simulink model "BenchmarkModel_Dynamic_TestCase"  (R2020a)
settings: Solver=ode45  StartTime=0.0  StopTime=5  RelTol=1e-3
undefined symbols (not defined in the file): Angle, D1, Delta, find_system, Magnitude
libraries: powerlib x91, powerlib_meascontrol x31, simulink x6, dspsrcs4 x3, dspsigops x2, sps_avr x1
(part 3 of 3)

== system BenchmarkModel_Dynamic_TestCase/VSI Converter1/Current Control/PLL & Park Transformation/Filter2 ==
  in : Inport
  Demux : Demux  Outputs=3
  Mux : Mux  Inputs=3
  Transfer Fcn1 : TransferFcn  Denominator=[1/(2*pi*Ft) 1]
  Transfer Fcn2 : TransferFcn  Denominator=[1/(2*pi*Ft) 1]
  Transfer Fcn3 : TransferFcn  Denominator=[1/(2*pi*Ft) 1]
  out : Outport  VectorParamsAs1DForOutWhenUnconnected=off
  wires:
  Mux/1 -> out/1
  in/1 -> Demux/1
  Transfer Fcn3/1 -> Mux/3
  Transfer Fcn2/1 -> Mux/2
  Transfer Fcn1/1 -> Mux/1
  Demux/3 -> Transfer Fcn3/1
  Demux/1 -> Transfer Fcn1/1
  Demux/2 -> Transfer Fcn2/1

== system BenchmarkModel_Dynamic_TestCase/VSI Converter1/Current Control/PLL & Park Transformation/Filter3 ==
  in : Inport
  Demux : Demux  Outputs=3
  Mux : Mux  Inputs=3
  Transfer Fcn1 : TransferFcn  Denominator=[1/(2*pi*Ft) 1]
  Transfer Fcn2 : TransferFcn  Denominator=[1/(2*pi*Ft) 1]
  Transfer Fcn3 : TransferFcn  Denominator=[1/(2*pi*Ft) 1]
  out : Outport  VectorParamsAs1DForOutWhenUnconnected=off
  wires:
  Demux/2 -> Transfer Fcn2/1
  Demux/1 -> Transfer Fcn1/1
  Demux/3 -> Transfer Fcn3/1
  Transfer Fcn1/1 -> Mux/1
  Transfer Fcn2/1 -> Mux/2
  Transfer Fcn3/1 -> Mux/3
  in/1 -> Demux/1
  Mux/1 -> out/1

== system BenchmarkModel_Dynamic_TestCase/VSI Converter1/Current Control/PLL & Park Transformation/MAF-PLL ==
  note: MAF
  Vabc : Inport
  Autoresettable integral theta : Subsystem
  Constant : Constant  Value=Non_limited_theta
  Demux9 : Demux  Outputs=2
  Divide : Product  Inputs=*/
  Gain : Gain  Gain=1/(2*pi)
  Gain1 : Gain  Gain=2*pi
  Gain2 : Gain  Gain=Ki_PLL
  Integrator : Integrator
  MAF : Subsystem
  MAF1 : Subsystem
  Proportional gain : Gain  Gain=Kp_PLL
  Selector : Selector  InputPortWidth=3  IndexOptions=Index vector (dialog)  Indices=[2 1]  OutputSizes=1
  Sum : Sum  Inputs=++|
  Sum2 : Sum  Inputs=++|
  Switch : Switch  Criteria=u2 > Threshold
  abc to dq3 : powerlib_meascontrol/Transformations/abc to dq0  Alignment=90 degrees behind phase A axis
  integration of pulse : Integrator  InitialCondition=initPhase*pi/180
  nominal frequency : Constant  Value=initFreq
  Estimated Theta : Outport  VectorParamsAs1DForOutWhenUnconnected=off
  Estimated Frequency : Outport  Port=2  VectorParamsAs1DForOutWhenUnconnected=off
  wires:
  Autoresettable integral theta/1(Out1) -> Switch/3
  Switch/1 -> abc to dq3/2, Estimated Theta/1  "Theta_o"
  Constant/1 -> Switch/2
  MAF1/1(Output) -> Divide/2
  MAF/1(Output) -> Divide/1
  Gain1/1 -> Sum2/1
  Gain/1 -> Estimated Frequency/1
  Demux9/1 -> MAF/1(Input)  "Vq"
  Demux9/2 -> MAF1/1(Input)  "Vd"
  Divide/1 -> Gain2/1, Proportional gain/1
  Proportional gain/1 -> Sum/2  "Delta_W_o"
  integration of pulse/1 -> Switch/1  "Theta_o"
  Vabc/1 -> abc to dq3/1
  Selector/1 -> Demux9/1  "Vq,Vd"
  nominal frequency/1 -> Gain1/1
  Sum/1 -> Gain/1, integration of pulse/1, Autoresettable integral theta/1(In1)  "W_o"
  abc to dq3/1 -> Selector/1
  Gain2/1 -> Integrator/1
  Integrator/1 -> Sum2/2
  Sum2/1 -> Sum/1

== system BenchmarkModel_Dynamic_TestCase/VSI Converter1/Current Control/PLL & Park Transformation/Park Capacitor Voltage ==
  note: PARK
  abc quantity : Inport
  f : Inport  Port=2
  Theta : Inport  Port=3
  Demux8 : Demux  Outputs=3
  Mag correction4 : Subsystem
  Phase correction4 : Subsystem
  Product : Product  Inputs=**
  Sum1 : Sum  Inputs=|+-
  Terminator7 : Terminator
  abc to dq7 : powerlib_meascontrol/Transformations/abc to dq0  Alignment=90 degrees behind phase A axis
  d quantity : Outport  VectorParamsAs1DForOutWhenUnconnected=off
  q quantity : Outport  Port=2  VectorParamsAs1DForOutWhenUnconnected=off
  wires:
  Phase correction4/1(Out1) -> Sum1/2
  f/1 -> Phase correction4/1(freq), Mag correction4/1(freq)
  abc quantity/1 -> Product/1
  Product/1 -> abc to dq7/1
  Mag correction4/1(Out1) -> Product/2
  Demux8/3 -> Terminator7/1
  Theta/1 -> Sum1/1
  Sum1/1 -> abc to dq7/2
  Demux8/2 -> q quantity/1  "q"
  Demux8/1 -> d quantity/1  "d"
  abc to dq7/1 -> Demux8/1

== system BenchmarkModel_Dynamic_TestCase/VSI Converter1/Current Control/PLL & Park Transformation/Park Current ==
  note: PARK
  abc quantity : Inport
  f : Inport  Port=2
  Theta : Inport  Port=3
  Demux8 : Demux  Outputs=3
  Mag correction4 : Subsystem
  Phase correction4 : Subsystem
  Product : Product  Inputs=**
  Sum1 : Sum  Inputs=|+-
  Terminator7 : Terminator
  abc to dq7 : powerlib_meascontrol/Transformations/abc to dq0  Alignment=90 degrees behind phase A axis
  d quantity : Outport  VectorParamsAs1DForOutWhenUnconnected=off
  q quantity : Outport  Port=2  VectorParamsAs1DForOutWhenUnconnected=off
  wires:
  Phase correction4/1(Out1) -> Sum1/2
  f/1 -> Phase correction4/1(freq), Mag correction4/1(freq)
  abc quantity/1 -> Product/1
  Product/1 -> abc to dq7/1
  Mag correction4/1(Out1) -> Product/2
  Demux8/3 -> Terminator7/1
  Theta/1 -> Sum1/1
  Sum1/1 -> abc to dq7/2
  Demux8/2 -> q quantity/1  "q"
  Demux8/1 -> d quantity/1  "d"
  abc to dq7/1 -> Demux8/1

== system BenchmarkModel_Dynamic_TestCase/VSI Converter1/Current Control/PLL & Park Transformation/Park Grid Voltage ==
  note: PARK
  abc quantity : Inport
  f : Inport  Port=2
  Theta : Inport  Port=3
  Demux8 : Demux  Outputs=3
  Mag correction4 : Subsystem
  Phase correction4 : Subsystem
  Product : Product  Inputs=**
  Sum1 : Sum  Inputs=|+-
  Terminator7 : Terminator
  abc to dq7 : powerlib_meascontrol/Transformations/abc to dq0  Alignment=90 degrees behind phase A axis
  d quantity : Outport  VectorParamsAs1DForOutWhenUnconnected=off
  q quantity : Outport  Port=2  VectorParamsAs1DForOutWhenUnconnected=off
  wires:
  abc to dq7/1 -> Demux8/1
  Demux8/1 -> d quantity/1  "d"
  Demux8/2 -> q quantity/1  "q"
  Sum1/1 -> abc to dq7/2
  Theta/1 -> Sum1/1
  Demux8/3 -> Terminator7/1
  Mag correction4/1(Out1) -> Product/2
  Product/1 -> abc to dq7/1
  abc quantity/1 -> Product/1
  f/1 -> Mag correction4/1(freq), Phase correction4/1(freq)
  Phase correction4/1(Out1) -> Sum1/2

== system BenchmarkModel_Dynamic_TestCase/VSI Converter1/Current Control/PLL & Park Transformation/concatenate//fase1 ==
  note: Vab
  note: Vbc
  note: Vca
  note: 3Va
  note: 3Vb
  note: 3Vc
  ab_bc_ca : Inport
  Add : Sum  Inputs=+-
  Add1 : Sum  Inputs=+-
  Add2 : Sum  Inputs=+-
  Demux : Demux  Outputs=3
  Gain : Gain  Gain=1/3
  Mux : Mux  Inputs=3
  a_b_c : Outport  VectorParamsAs1DForOutWhenUnconnected=off
  wires:
  Demux/2 -> Add1/1, Add2/2
  Demux/3 -> Add/2, Add2/1
  Demux/1 -> Add1/2, Add/1
  Gain/1 -> a_b_c/1
  Mux/1 -> Gain/1
  Add2/1 -> Mux/3
  Add1/1 -> Mux/2
  Add/1 -> Mux/1
  ab_bc_ca/1 -> Demux/1

== system BenchmarkModel_Dynamic_TestCase/VSI Converter1/Current Control/PLL & Park Transformation/concatenate//fase2 ==
  note: 3Vc
  note: 3Vb
  note: 3Va
  note: Vca
  note: Vbc
  note: Vab
  ab_bc_ca : Inport
  Add : Sum  Inputs=+-
  Add1 : Sum  Inputs=+-
  Add2 : Sum  Inputs=+-
  Demux : Demux  Outputs=3
  Gain : Gain  Gain=1/3
  Mux : Mux  Inputs=3
  a_b_c : Outport  VectorParamsAs1DForOutWhenUnconnected=off
  wires:
  ab_bc_ca/1 -> Demux/1
  Add/1 -> Mux/1
  Add1/1 -> Mux/2
  Add2/1 -> Mux/3
  Mux/1 -> Gain/1
  Gain/1 -> a_b_c/1
  Demux/1 -> Add/1, Add1/2
  Demux/3 -> Add2/1, Add/2
  Demux/2 -> Add2/2, Add1/1

== system BenchmarkModel_Dynamic_TestCase/VSI Converter1/Current Control/Qref --> Iqref/Parameter ==
  Constant8 : Constant  Value=1e-3
  Constant9 : Constant  Value=Cf
  Mux1 : Mux  Inputs=2
  Parameters : Outport  VectorParamsAs1DForOutWhenUnconnected=off
  wires:
  Mux1/1 -> Parameters/1
  Constant8/1 -> Mux1/1
  Constant9/1 -> Mux1/2

== system BenchmarkModel_Dynamic_TestCase/VSI Converter1/Current Control/Qref --> Iqref/Vc ==
  VCd : Inport
  VCq : Inport  Port=2
  Complex to Magnitude-Angle3 : ComplexToMagnitudeAngle
  Constant12 : Constant  Value=sqrt(2)
  Divide5 : Product  Inputs=*/
  Real-Imag to Complex3 : RealImagToComplex
  Terminator6 : Terminator
  Vc_rms : Outport  VectorParamsAs1DForOutWhenUnconnected=off
  wires:
  Real-Imag to Complex3/1 -> Complex to Magnitude-Angle3/1
  Complex to Magnitude-Angle3/2 -> Terminator6/1
  VCd/1 -> Real-Imag to Complex3/1
  VCq/1 -> Real-Imag to Complex3/2
  Constant12/1 -> Divide5/2
  Complex to Magnitude-Angle3/1 -> Divide5/1
  Divide5/1 -> Vc_rms/1

== system BenchmarkModel_Dynamic_TestCase/Subsystem/Three-Phase Tap Changer Transformer Pn MVA, Up // Us kV/Tap Changer Control/Edge Detector/NEGATIVE Edge ==
  IN : Inport
  IN previous : Inport  Port=2
  Enable : EnablePort  PropagateVarSize=During execution
  Relational Operator1 : RelationalOperator  Operator=>  RndMeth=Nearest  InputSameDT=on
  OUT : Outport  VectorParamsAs1DForOutWhenUnconnected=off
  wires:
  Relational Operator1/1 -> OUT/1
  IN previous/1 -> Relational Operator1/1
  IN/1 -> Relational Operator1/2

== system BenchmarkModel_Dynamic_TestCase/Subsystem/Three-Phase Tap Changer Transformer Pn MVA, Up // Us kV/Tap Changer Control/Edge Detector/POSITIVE Edge ==
  IN : Inport
  IN previous : Inport  Port=2
  Enable : EnablePort  PropagateVarSize=During execution
  Relational Operator1 : RelationalOperator  Operator=>  RndMeth=Nearest  InputSameDT=on
  OUT : Outport  VectorParamsAs1DForOutWhenUnconnected=off
  wires:
  Relational Operator1/1 -> OUT/1
  IN previous/1 -> Relational Operator1/2
  IN/1 -> Relational Operator1/1

== system BenchmarkModel_Dynamic_TestCase/VSI Converter1/Current Control/PLL & Park Transformation/MAF-PLL/Autoresettable integral theta ==
  In1 : Inport
  Add : Sum  Inputs=+-
  Constant : Constant  Value=2*pi
  Divide : Product  Inputs=*/  OutDataTypeStr=int32  SaturateOnIntegerOverflow=on
  Gain : Gain  Gain=2*pi
  Integrator : Integrator  InitialCondition=initPhase*pi/180
  Out1 : Outport  VectorParamsAs1DForOutWhenUnconnected=off
  wires:
  Add/1 -> Out1/1
  Gain/1 -> Add/2
  Divide/1 -> Gain/1
  Constant/1 -> Divide/2
  In1/1 -> Integrator/1
  Integrator/1 -> Divide/1, Add/1

== system BenchmarkModel_Dynamic_TestCase/VSI Converter1/Current Control/PLL & Park Transformation/MAF-PLL/MAF ==
  Input : Inport
  Delay of Tw : TransportDelay  DelayTime=Tw
  Gain : Gain  Gain=1/Tw
  Integrator2 : Integrator
  Sum : Sum  Inputs=+-
  Output : Outport  VectorParamsAs1DForOutWhenUnconnected=off
  wires:
  Integrator2/1 -> Output/1
  Delay of Tw/1 -> Sum/2
  Input/1 -> Sum/1, Delay of Tw/1
  Sum/1 -> Gain/1
  Gain/1 -> Integrator2/1

== system BenchmarkModel_Dynamic_TestCase/VSI Converter1/Current Control/PLL & Park Transformation/MAF-PLL/MAF1 ==
  Input : Inport
  Delay of Tw : TransportDelay  DelayTime=Tw
  Gain : Gain  Gain=1/Tw
  Integrator2 : Integrator  InitialCondition=326
  Sum : Sum  Inputs=+-
  Output : Outport  VectorParamsAs1DForOutWhenUnconnected=off
  wires:
  Gain/1 -> Integrator2/1
  Sum/1 -> Gain/1
  Input/1 -> Delay of Tw/1, Sum/1
  Delay of Tw/1 -> Sum/2
  Integrator2/1 -> Output/1

== system BenchmarkModel_Dynamic_TestCase/VSI Converter1/Current Control/PLL & Park Transformation/Park Capacitor Voltage/Mag correction4 ==
  freq : Inport
  Complex to Magnitude-Angle : ComplexToMagnitudeAngle
  Divide5 : Product  Inputs=**/
  Real-Imag to Complex : RealImagToComplex
  Terminator : Terminator
  w10 : Constant  Value=2*pi*Ft
  w11 : Constant
  w9 : Constant  Value=2*pi
  Out1 : Outport  VectorParamsAs1DForOutWhenUnconnected=off
  wires:
  freq/1 -> Divide5/2
  w10/1 -> Divide5/3
  w9/1 -> Divide5/1
  Divide5/1 -> Real-Imag to Complex/2
  Complex to Magnitude-Angle/2 -> Terminator/1
  Complex to Magnitude-Angle/1 -> Out1/1
  w11/1 -> Real-Imag to Complex/1
  Real-Imag to Complex/1 -> Complex to Magnitude-Angle/1

== system BenchmarkModel_Dynamic_TestCase/VSI Converter1/Current Control/PLL & Park Transformation/Park Capacitor Voltage/Phase correction4 ==
  freq : Inport
  Divide2 : Product  Inputs=**/
  Trigonometric Function1 : Trigonometry  Operator=atan
  w3 : Constant  Value=2*pi
  w4 : Constant  Value=2*pi*Ft
  Out1 : Outport  VectorParamsAs1DForOutWhenUnconnected=off
  wires:
  Trigonometric Function1/1 -> Out1/1
  Divide2/1 -> Trigonometric Function1/1
  freq/1 -> Divide2/2
  w4/1 -> Divide2/3
  w3/1 -> Divide2/1

== system BenchmarkModel_Dynamic_TestCase/VSI Converter1/Current Control/PLL & Park Transformation/Park Current/Mag correction4 ==
  freq : Inport
  Complex to Magnitude-Angle : ComplexToMagnitudeAngle
  Divide5 : Product  Inputs=**/
  Real-Imag to Complex : RealImagToComplex
  Terminator : Terminator
  w10 : Constant  Value=2*pi*Ft
  w11 : Constant
  w9 : Constant  Value=2*pi
  Out1 : Outport  VectorParamsAs1DForOutWhenUnconnected=off
  wires:
  freq/1 -> Divide5/2
  w10/1 -> Divide5/3
  w9/1 -> Divide5/1
  Divide5/1 -> Real-Imag to Complex/2
  Complex to Magnitude-Angle/2 -> Terminator/1
  Complex to Magnitude-Angle/1 -> Out1/1
  w11/1 -> Real-Imag to Complex/1
  Real-Imag to Complex/1 -> Complex to Magnitude-Angle/1

== system BenchmarkModel_Dynamic_TestCase/VSI Converter1/Current Control/PLL & Park Transformation/Park Current/Phase correction4 ==
  freq : Inport
  Divide2 : Product  Inputs=**/
  Trigonometric Function1 : Trigonometry  Operator=atan
  w3 : Constant  Value=2*pi
  w4 : Constant  Value=2*pi*Ft
  Out1 : Outport  VectorParamsAs1DForOutWhenUnconnected=off
  wires:
  Trigonometric Function1/1 -> Out1/1
  Divide2/1 -> Trigonometric Function1/1
  freq/1 -> Divide2/2
  w4/1 -> Divide2/3
  w3/1 -> Divide2/1

== system BenchmarkModel_Dynamic_TestCase/VSI Converter1/Current Control/PLL & Park Transformation/Park Grid Voltage/Mag correction4 ==
  freq : Inport
  Complex to Magnitude-Angle : ComplexToMagnitudeAngle
  Divide5 : Product  Inputs=**/
  Real-Imag to Complex : RealImagToComplex
  Terminator : Terminator
  w10 : Constant  Value=2*pi*Ft
  w11 : Constant
  w9 : Constant  Value=2*pi
  Out1 : Outport  VectorParamsAs1DForOutWhenUnconnected=off
  wires:
  Real-Imag to Complex/1 -> Complex to Magnitude-Angle/1
  w11/1 -> Real-Imag to Complex/1
  Complex to Magnitude-Angle/1 -> Out1/1
  Complex to Magnitude-Angle/2 -> Terminator/1
  Divide5/1 -> Real-Imag to Complex/2
  w9/1 -> Divide5/1
  w10/1 -> Divide5/3
  freq/1 -> Divide5/2

== system BenchmarkModel_Dynamic_TestCase/VSI Converter1/Current Control/PLL & Park Transformation/Park Grid Voltage/Phase correction4 ==
  freq : Inport
  Divide2 : Product  Inputs=**/
  Trigonometric Function1 : Trigonometry  Operator=atan
  w3 : Constant  Value=2*pi
  w4 : Constant  Value=2*pi*Ft
  Out1 : Outport  VectorParamsAs1DForOutWhenUnconnected=off
  wires:
  w3/1 -> Divide2/1
  w4/1 -> Divide2/3
  freq/1 -> Divide2/2
  Divide2/1 -> Trigonometric Function1/1
  Trigonometric Function1/1 -> Out1/1

== matlab function BenchmarkModel_Dynamic_TestCase/VSI Converter1/Current Control/Qref --> Iqref/Filter Compensation ==
  data: f input; Vc input; Param input; Qc output
function Qc  = fcn(f,Vc,Param)

Rf = Param(1);
Cf = Param(2);
W = 2*pi*f;

Qc = 3*imag( i*W*Cf*Vc^2  / (i*W*Rf*Cf + 1) );

[Qc];

== matlab function BenchmarkModel_Dynamic_TestCase/VSI Converter1/Saturation ==
  data: SAT output; Vd input; Vq input; Vd_out output; Vq_out output; Vdc input
function [SAT,Vd_out,Vq_out] = W_Sat(Vd,Vq,Vdc)
module=sqrt(Vd^2+Vq^2);
Vlimit=Vdc*0.997;

if(module>=Vlimit)
    Vd_out = Vd*Vlimit / module;
    Vq_out = Vq*Vlimit / module;
    SAT = true;
else
    Vd_out = Vd;
    Vq_out = Vq;
    SAT = false;
end

[SAT,Vd_out,Vq_out];
